simulink model "NL_2DOF"  (R2019b)
settings: Solver=VariableStepAuto  StartTime=0.0  StopTime=200  RelTol=1e-3
InitFcn:
  | load("parameters.mat");
  | load("Coefficients.mat");
undefined symbols (not defined in the file): Dm2, Dt, g, Jp, Jy, k_pitch_, k_py, k_yaw, k_yp, Mb, Pitch, w_ramp_0N, w_ramp_0P, w_ramp_1N, w_ramp_1P, Yaw
settings Model: Creator=laptop  LastModifiedBy=lbend

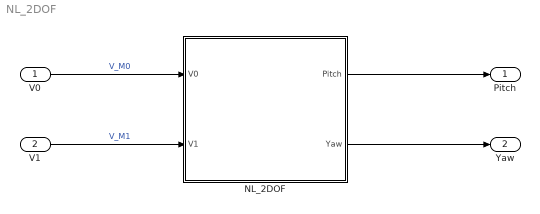
== system NL_2DOF ==
  V0 : Inport
  V1 : Inport  Port=2
  NL_2DOF : Subsystem  mask{YawButton=Yaw Movement, PitchButton=Pitch Movement}
      mask prompts: YawButton "YAW doF"; PitchButton "PITCH doF"
      mask TypeOptions YawButton: Yaw Movement | Yaw Locked
      mask Callback YawButton:
      | y = get_param(gcbh,'YawButton');
      | 
      | switch y
      |     case 'Yaw Movement'
      |         Yaw = 1;
      |     case 'Yaw Locked'
      |         Yaw = 0;
      | end
      | 
      | assignin("base","Yaw",Yaw);
      mask TypeOptions PitchButton: Pitch Movement | Pitch Locked
      mask Callback PitchButton:
      | p = get_param(gcbh,'PitchButton');
      | 
      | switch p
      |     case 'Pitch Movement'
      |         Pitch = 1;
      |     case 'Pitch Locked'
      |         Pitch = 0;
      | end
      | 
      | assignin("base","Pitch", Pitch);
      mask DialogControl DescGroupVar Prompt: Degrees of Freedom
      mask DialogControl DescTextVar Prompt: Here you can select the working mode for the model
      mask Display: image('C:\Users\lbend\OneDrive - Politecnico di Milano\Root Locos\Reports\Photos&Images\2doF.png');
  Pitch : Outport
  Yaw : Outport  Port=2
  wires:
  V0/1 -> NL_2DOF/1(V0)  "V_M0"
  V1/1 -> NL_2DOF/2(V1)  "V_M1"
  NL_2DOF/1(Pitch) -> Pitch/1
  NL_2DOF/2(Yaw) -> Yaw/1

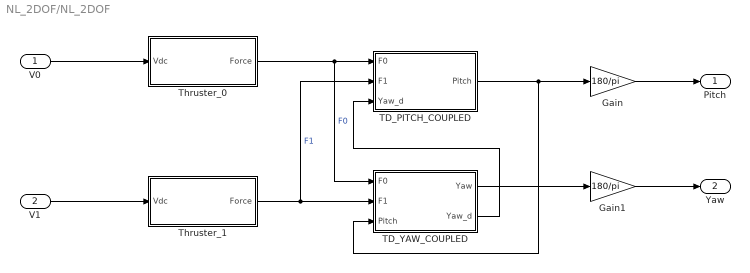
== system NL_2DOF/NL_2DOF ==
  V0 : Inport
  V1 : Inport  Port=2
  Gain : Gain  Gain=180/pi
  Gain1 : Gain  Gain=180/pi
  TD_PITCH_COUPLED : Subsystem
  TD_YAW_COUPLED : Subsystem
  Thruster_0 : Subsystem
  "Thruster_1 " : Subsystem
  Pitch : Outport
  Yaw : Outport  Port=2
  wires:
  V1/1 -> "Thruster_1 "/1(Vdc)
  Gain/1 -> Pitch/1
  V0/1 -> Thruster_0/1(Vdc)
  TD_YAW_COUPLED/1(Yaw) -> Gain1/1
  Gain1/1 -> Yaw/1
  TD_PITCH_COUPLED/1(Pitch) -> TD_YAW_COUPLED/3(Pitch), Gain/1
  "Thruster_1 "/1(Force) -> TD_PITCH_COUPLED/2("F1 "), TD_YAW_COUPLED/2(F1)  "F1"
  Thruster_0/1(Force) -> TD_YAW_COUPLED/1(F0), TD_PITCH_COUPLED/1(F0)  "F0"
  TD_YAW_COUPLED/2(Yaw_d) -> TD_PITCH_COUPLED/3(Yaw_d)

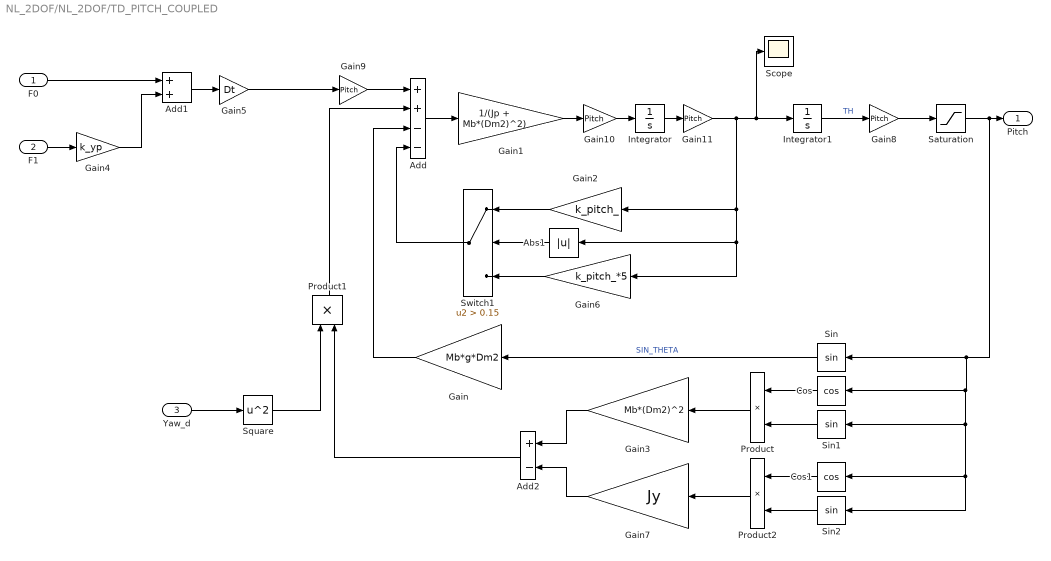
== system NL_2DOF/NL_2DOF/TD_PITCH_COUPLED ==
  F0 : Inport
  "F1 " : Inport  Port=2
  Yaw_d : Inport  Port=3
  Abs1 : Abs
  Add : Sum  Inputs=++--
  Add1 : Sum
  Add2 : Sum  Inputs=+-
  Cos : Trigonometry  Operator=cos
  Cos1 : Trigonometry  Operator=cos
  Gain : Gain  Gain=Mb*g*Dm2
  Gain1 : Gain  Gain=1/(Jp + Mb*(Dm2)^2)
  Gain{8..11} (4 alike) : Gain  Gain=Pitch
  Gain2 : Gain  Gain=k_pitch_
  Gain3 : Gain  Gain=Mb*(Dm2)^2
  Gain4 : Gain  Gain=k_yp
  Gain5 : Gain  Gain=Dt
  Gain6 : Gain  Gain=k_pitch_*5
  Gain7 : Gain  Gain=Jy
  Integrator : Integrator
  Integrator1 : Integrator
  Product : Product
  Product1 : Product
  Product2 : Product
  Saturation : Saturate  UpperLimit=0.93  LowerLimit=-0.93  LinearizeAsGain=off
  Scope : Scope
  Sin : Trigonometry
  Sin1 : Trigonometry
  Sin2 : Trigonometry
  Square : Math  Operator=square  SignedPower=off  SaturateOnIntegerOverflow=on
  Switch1 : Switch  Criteria=u2 > Threshold  Threshold=0.15  RndMeth=Simplest
  Pitch : Outport
  wires:
  Sin/1 -> Gain/1  "SIN_THETA"
  Add/1 -> Gain1/1
  Gain1/1 -> Gain10/1
  Gain5/1 -> Gain9/1
  F0/1 -> Add1/1
  "F1 "/1 -> Gain4/1
  Gain4/1 -> Add1/2
  Add1/1 -> Gain5/1
  Sin1/1 -> Product/2
  Cos/1 -> Product/1
  Product/1 -> Gain3/1
  Gain/1 -> Add/3
  Yaw_d/1 -> Square/1
  Product1/1 -> Add/2
  Square/1 -> Product1/1
  Gain3/1 -> Add2/1
  Add2/1 -> Product1/2
  Gain7/1 -> Add2/2
  Cos1/1 -> Product2/1
  Saturation/1 -> Pitch/1, Cos1/1, Sin2/1, Sin1/1, Cos/1, Sin/1
  Sin2/1 -> Product2/2
  Product2/1 -> Gain7/1
  Gain6/1 -> Switch1/3
  Integrator/1 -> Gain11/1
  Abs1/1 -> Switch1/2
  Switch1/1 -> Add/4
  Gain2/1 -> Switch1/1
  Integrator1/1 -> Gain8/1  "TH"
  Gain8/1 -> Saturation/1
  Gain9/1 -> Add/1
  Gain10/1 -> Integrator/1
  Gain11/1 -> Gain6/1, Abs1/1, Gain2/1, Scope/1, Integrator1/1

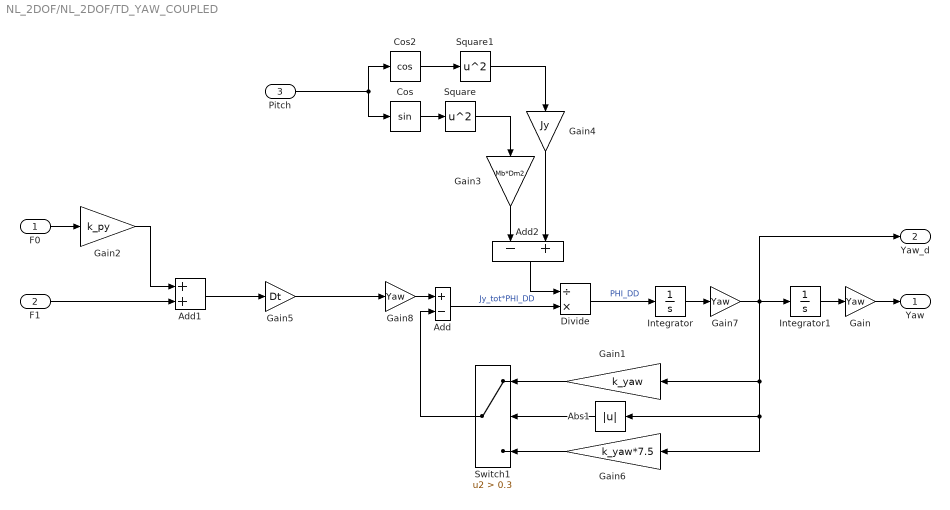
== system NL_2DOF/NL_2DOF/TD_YAW_COUPLED ==
  F0 : Inport
  F1 : Inport  Port=2
  Pitch : Inport  Port=3
  Abs1 : Abs
  Add : Sum  Inputs=+-
  Add1 : Sum
  Add2 : Sum  Inputs=-+
  Cos : Trigonometry
  Cos2 : Trigonometry  Operator=cos
  Divide : Product  Inputs=/*
  Gain : Gain  Gain=Yaw
  Gain1 : Gain  Gain=k_yaw
  Gain2 : Gain  Gain=k_py
  Gain3 : Gain  Gain=Mb*Dm2
  Gain4 : Gain  Gain=Jy
  Gain5 : Gain  Gain=Dt
  Gain6 : Gain  Gain=k_yaw*7.5
  Gain7 : Gain  Gain=Yaw
  Gain8 : Gain  Gain=Yaw
  Integrator : Integrator
  Integrator1 : Integrator
  Square : Math  Operator=square  SignedPower=off  SaturateOnIntegerOverflow=on
  Square1 : Math  Operator=square  SignedPower=off  SaturateOnIntegerOverflow=on
  Switch1 : Switch  Criteria=u2 > Threshold  Threshold=0.3
  Yaw : Outport
  Yaw_d : Outport  Port=2
  wires:
  Gain2/1 -> Add1/1
  Integrator/1 -> Gain7/1
  Add/1 -> Divide/2  "Jy_tot*PHI_DD"
  Divide/1 -> Integrator/1  "PHI_DD"
  F1/1 -> Add1/2
  F0/1 -> Gain2/1
  Integrator1/1 -> Gain/1
  Add1/1 -> Gain5/1
  Gain5/1 -> Gain8/1
  Pitch/1 -> Cos/1, Cos2/1
  Cos/1 -> Square/1
  Square/1 -> Gain3/1
  Gain3/1 -> Add2/1
  Gain4/1 -> Add2/2
  Cos2/1 -> Square1/1
  Add2/1 -> Divide/1
  Gain1/1 -> Switch1/1
  Abs1/1 -> Switch1/2
  Switch1/1 -> Add/2
  Gain6/1 -> Switch1/3
  Square1/1 -> Gain4/1
  Gain/1 -> Yaw/1
  Gain7/1 -> Yaw_d/1, Integrator1/1, Abs1/1, Gain6/1, Gain1/1
  Gain8/1 -> Add/1

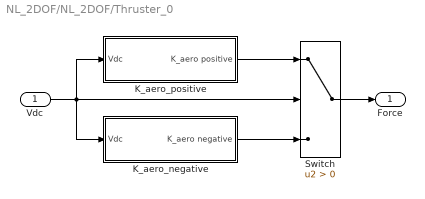
== system NL_2DOF/NL_2DOF/Thruster_0 ==
  Vdc : Inport
  K_aero_negative : Subsystem
  K_aero_positive : Subsystem
  Switch : Switch  Criteria=u2 > Threshold
  Force : Outport
  wires:
  Switch/1 -> Force/1
  K_aero_positive/1(K_aero positive) -> Switch/1
  Vdc/1 -> K_aero_positive/1(Vdc), K_aero_negative/1(Vdc), Switch/2
  K_aero_negative/1(K_aero negative) -> Switch/3

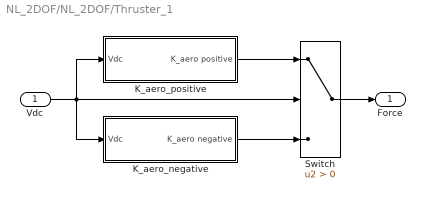
== system NL_2DOF/NL_2DOF/Thruster_1  ==
  Vdc : Inport
  K_aero_negative : Subsystem
  K_aero_positive : Subsystem
  Switch : Switch  Criteria=u2 > Threshold
  Force : Outport
  wires:
  Switch/1 -> Force/1
  K_aero_positive/1(K_aero positive) -> Switch/1
  Vdc/1 -> K_aero_negative/1(Vdc), Switch/2, K_aero_positive/1(Vdc)
  K_aero_negative/1(K_aero negative) -> Switch/3

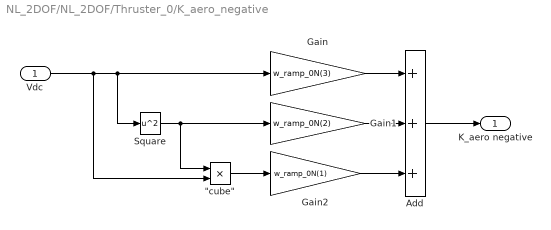
== system NL_2DOF/NL_2DOF/Thruster_0/K_aero_negative ==
  Vdc : Inport
  "\"cube\"" : Product  Inputs=**
  Add : Sum  Inputs=+++
  Gain : Gain  Gain=w_ramp_0N(3)
  Gain1 : Gain  Gain=w_ramp_0N(2)
  Gain2 : Gain  Gain=w_ramp_0N(1)
  Square : Math  Operator=square  SignedPower=off  SaturateOnIntegerOverflow=on
  K_aero negative : Outport
  wires:
  Vdc/1 -> "\"cube\""/2, Square/1, Gain/1
  Gain/1 -> Add/1
  Square/1 -> "\"cube\""/1, Gain1/1
  Gain1/1 -> Add/2
  Gain2/1 -> Add/3
  "\"cube\""/1 -> Gain2/1
  Add/1 -> K_aero negative/1

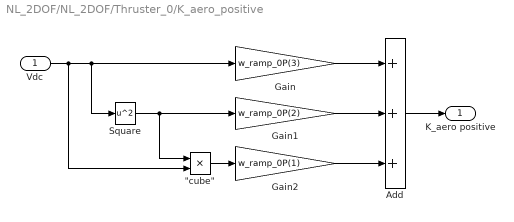
== system NL_2DOF/NL_2DOF/Thruster_0/K_aero_positive ==
  Vdc : Inport
  "\"cube\"" : Product  Inputs=**
  Add : Sum  Inputs=+++
  Gain : Gain  Gain=w_ramp_0P(3)
  Gain1 : Gain  Gain=w_ramp_0P(2)
  Gain2 : Gain  Gain=w_ramp_0P(1)
  Square : Math  Operator=square  SignedPower=off  SaturateOnIntegerOverflow=on
  K_aero positive : Outport
  wires:
  Vdc/1 -> Gain/1, Square/1, "\"cube\""/2
  Add/1 -> K_aero positive/1
  Gain/1 -> Add/1
  Square/1 -> "\"cube\""/1, Gain1/1
  Gain1/1 -> Add/2
  "\"cube\""/1 -> Gain2/1
  Gain2/1 -> Add/3

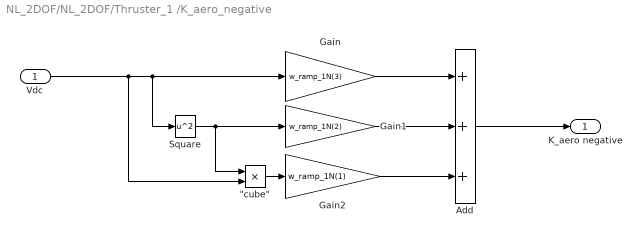
== system NL_2DOF/NL_2DOF/Thruster_1 /K_aero_negative ==
  Vdc : Inport
  "\"cube\"" : Product  Inputs=**
  Add : Sum  Inputs=+++
  Gain : Gain  Gain=w_ramp_1N(3)
  Gain1 : Gain  Gain=w_ramp_1N(2)
  Gain2 : Gain  Gain=w_ramp_1N(1)
  Square : Math  Operator=square  SignedPower=off  SaturateOnIntegerOverflow=on
  K_aero negative : Outport
  wires:
  Vdc/1 -> "\"cube\""/2, Square/1, Gain/1
  Gain/1 -> Add/1
  Square/1 -> "\"cube\""/1, Gain1/1
  Gain1/1 -> Add/2
  Gain2/1 -> Add/3
  "\"cube\""/1 -> Gain2/1
  Add/1 -> K_aero negative/1

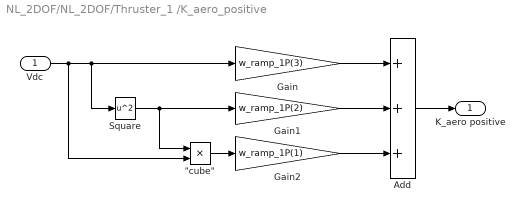
== system NL_2DOF/NL_2DOF/Thruster_1 /K_aero_positive ==
  Vdc : Inport
  "\"cube\"" : Product  Inputs=**
  Add : Sum  Inputs=+++
  Gain : Gain  Gain=w_ramp_1P(3)
  Gain1 : Gain  Gain=w_ramp_1P(2)
  Gain2 : Gain  Gain=w_ramp_1P(1)
  Square : Math  Operator=square  SignedPower=off  SaturateOnIntegerOverflow=on
  K_aero positive : Outport
  wires:
  Vdc/1 -> Gain/1, Square/1, "\"cube\""/2
  Add/1 -> K_aero positive/1
  Gain/1 -> Add/1
  Square/1 -> "\"cube\""/1, Gain1/1
  Gain1/1 -> Add/2
  "\"cube\""/1 -> Gain2/1
  Gain2/1 -> Add/3
